simulink library "BUS_OUT"  (R2018b)
settings: Solver=VariableStepAuto  StartTime=0.0  StopTime=10.0  RelTol=1e-3
settings Model: Creator=Alexander Koch  LastModifiedBy=ga69qig
settings SFSimCC: SimUseLocalCustomCode=off
settings RTWCC: RTWUseLocalCustomCode=off
settings CodeAppCC: StateflowObjectComments=on

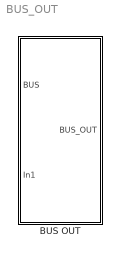
== system BUS_OUT ==
  BUS OUT : Subsystem  mask{NumberofInputs=1, NameSys='Subsystem'}
      mask prompts: NumberofInputs "Numper of costum inputs"; NameSys "Name of Bus Subsystem"
      mask help:
      | <Author> Alexander Koch, Benedikt Danquah based on Stefan Müller [1], Stephan Rohr [2]  </Author>
      |
      | <Date> 02/05/2017</Date>
      |
      | <Description>
      | Automated BUS Out Block for the Bus System. Allows to enter the Number of costum inputs and the name of the bus system. After entering the parameters the required amout of Inputs are built and connected to the Bus Creator. The signal names that are connected to the inputs In1, ..., InN are automatically adopted at the Bus signal names and can be found in the Bus under the name of the Bus Subsystem. If the signal (line) to the Inport has no name, the name of the previous blocks outport is taken. If this is not possible, the name if the previous block is taken for the Bus signal name.
      |
      | Additional, there are two buttons. The Refresh Input Names refreshes all Input Names. This is required if signal names are changed or signals are connected for the first time. To build a new system or if another Subsystem is added between existing subsystems, the Refresh Bus Selector is required at every subsystem that is calculated after the new subsystem.
      |
      | The Block automaticlly disconnects the link to the library block after opening the first time
      | </Description>
      mask init:
      | BusRefreshInputs()
      settings: OpenFcn=|
      | set_param(gcb(),'LinkStatus','none')
      | open_system(gcb(),'mask')
      mask Help:
      | <Parameters>
      | Number of costum inputs [-]
      | Name of Bus Subsystem ['abc']
      | </Parameters>
      | 
      | <Inputs>
      | Bus [Bus]
      | In1 [ ]
      | </Inputs>
      | 
      | <Outputs>
      | Bus [Bus]
      | </Outputs>
      | 
      | <Sources>
      | [1] S. Mueller, S. Rohr, W. Schmid, and M. Lienkamp, “Analysing the Influence of Driver Behaviour and Tuning Measures on Battery Aging and Residual Value of Electric Vehicles,” in Proc. EVS30 Symposium, Stuttgart, 2017, pp. 1–12.
      | [2] S. Rohr, “Technisch-wirtschaftliche Analyse des Zweitnutzungs- potentials von Lithium-Ionen-Traktionsbatterien,” Dissertation, Institute of Automotive Technology, Technical University Munich, Munich, 2018.
      | </Sources>
      mask DialogControl Container4 Prompt: Documentation:
      mask DialogControl Control4 Prompt: %<MaskHelp>
      mask DialogControl Container3 Prompt: Refresh
      mask DialogControl RefreshInputNames Prompt: Refresh Input Names
      mask DialogControl RefreshInputNames Callback: BusRefreshLineNames()
      mask DialogControl RefreshBusSelector Prompt: Refresh Bus Selector
      mask DialogControl RefreshBusSelector Callback: BusRefreshBusSelector()

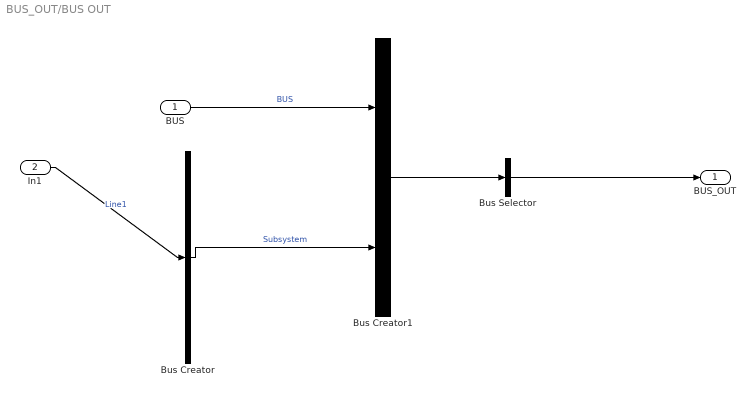
== system BUS_OUT/BUS OUT ==
  BUS : Inport
  In1 : Inport  Port=2
  Bus Creator : BusCreator  Inputs=NumberofInputs
  Bus Creator1 : BusCreator  Inputs=2
  Bus Selector : BusSelector  OutputSignals=Subsystem,BUS  OutputAsBus=on
  BUS_OUT : Outport
  wires:
  Bus Selector/1 -> BUS_OUT/1
  Bus Creator/1 -> Bus Creator1/2  "Subsystem"
  BUS/1 -> Bus Creator1/1  "BUS"
  Bus Creator1/1 -> Bus Selector/1
  In1/1 -> Bus Creator/1  "Line1"
